simulink model "prob4"  (R2020b)
settings: Solver=VariableStepAuto  StartTime=0.0  StopTime=10.0  RelTol=1e-3
model workspace (MAT data in the model file):
  k1 = Simulink.Parameter
  k1.Value = 0.4
  k1.DataType = 'auto'
  k1.Dimensions = [1 1]
  k2 = Simulink.Parameter
  k2.Value = 0.5
  k2.DataType = 'auto'
  k2.Dimensions = [1 1]
  k3 = Simulink.Parameter
  k3.Value = 0.25
  k3.DataType = 'auto'
  k3.Dimensions = [1 1]
settings Model: Creator=Admin  LastModifiedBy=Admin

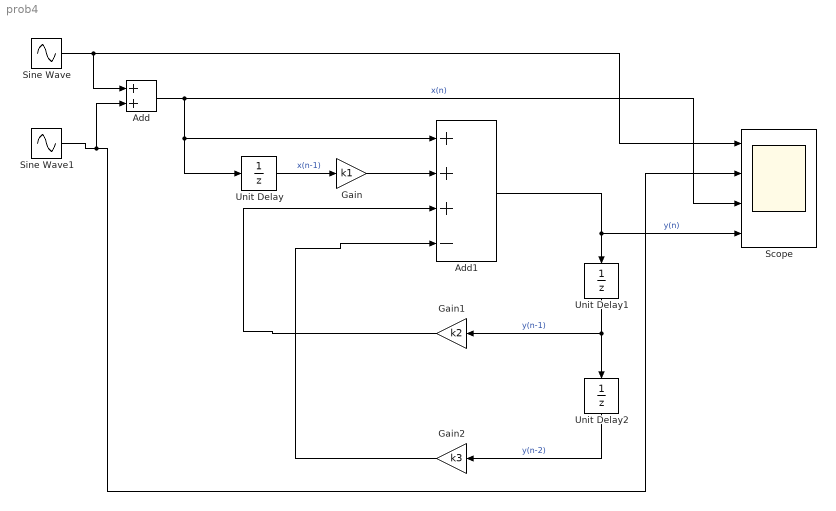
== system prob4 ==
  Add : Sum
  Add1 : Sum  Inputs=+++-
  Gain : Gain  Gain=k1
  Gain1 : Gain  Gain=k2
  Gain2 : Gain  Gain=k3
  Scope : Scope  NumInputPorts=4
  Sine Wave : Sin  SampleTime=0
  Sine Wave1 : Sin  Frequency=50  SampleTime=0
  Unit Delay : UnitDelay  SampleTime=-1  HasFrameUpgradeWarning=on
  Unit Delay1 : UnitDelay  SampleTime=-1  HasFrameUpgradeWarning=on
  Unit Delay2 : UnitDelay  SampleTime=-1  HasFrameUpgradeWarning=on
  wires:
  Sine Wave/1 -> Add/1, Scope/1
  Sine Wave1/1 -> Add/2, Scope/2
  Add/1 -> Add1/1, Unit Delay/1, Scope/3  "x(n)"
  Add1/1 -> Scope/4, Unit Delay1/1  "y(n)"
  Unit Delay1/1 -> Gain1/1, Unit Delay2/1  "y(n-1)"
  Unit Delay2/1 -> Gain2/1  "y(n-2)"
  Gain/1 -> Add1/2
  Unit Delay/1 -> Gain/1  "x(n-1)"
  Gain1/1 -> Add1/3
  Gain2/1 -> Add1/4
